simulink model "simulation"  (R2023a)
settings: Solver=VariableStepAuto  StartTime=0.0  StopTime=inf  RelTol=1e-3
values from neighbouring files (symbols this model uses):
  C_d = 0.1    [sim_script.m]
  C_l = 0.2    [parameters.m]
  fins_max_pos = deg2rad(15)    [parameters.m]
  fins_max_vel = deg2rad(180)    [parameters.m]
  g = 9.81    [parameters.m]    (also in sim_script.m)
  J_r = 0.000014703    (= 1.4703e-05)    [parameters.m]
  J_xx = 0.000834380    (= 0.00083438)    [parameters.m]
  J_yy = 0.000827389    [parameters.m]
  J_zz = 0.000150260    (= 0.00015026)    [parameters.m]
  K = lqr(A, B, Q, R)    [parameters.m]    (also in sim_script.m = lqr(A, B, Q, R, 0))
  K_t = 3.85756    [parameters.m]
  K_tau = 0.04249    [parameters.m]
  K_w = 0.0000014188    (= 1.4188e-06)    [parameters.m]    (also in sim_script.m = 1400)
  l = 0.04581 + 0.00625    (= 0.05206)    [parameters.m]    (also in sim_script.m = 0.1)
  m = 0.27765    [parameters.m]    (also in sim_script.m = 1)
  measurement_dt = 1/measurement_freq    (= 0.01)    [parameters.m]
  operating_point = [ ... (first row only)    [parameters.m]
  r = 0.06575    [parameters.m]    (also in sim_script.m = 0.05)
  variance_acc = 0.01    [parameters.m]
  variance_dst = 0.01    [parameters.m]
  variance_gyr = 0.01    [parameters.m]
  variance_mag = 0.01    [parameters.m]
undefined symbols (not defined in the file or in its folder): Discrete, throttle_max_rate, Time
libraries: sharedtransform x6, vrlib x4, commchan3 x4, matrix_library x2, shared6dof x1, ctrlSharedLib x1, sharedTrackingLibrary x1
settings Model: SimulationMode=accelerator  Creator=emozdzen  LastModifiedBy=emozdzen

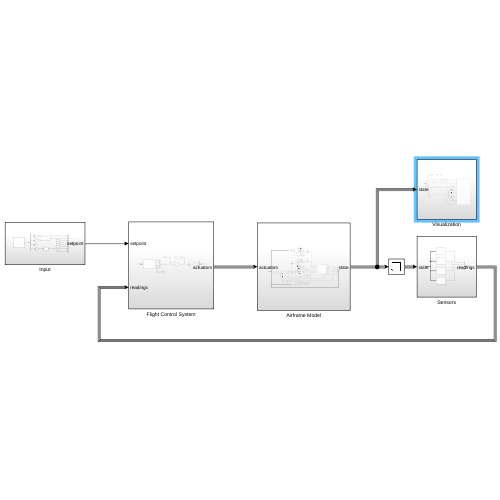
[thumbnail: Simulink's stored preview of the top-level diagram]
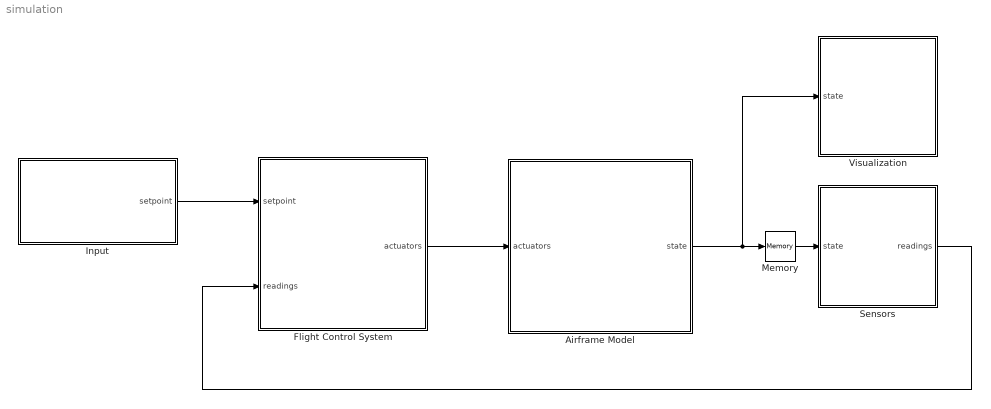
== system simulation ==
  Airframe Model : Subsystem
  Flight Control System : Subsystem
  Input : Subsystem
  Memory : Memory
  Sensors : Subsystem
  Visualization : Subsystem
  wires:
  Flight Control System/1(actuators) -> Airframe Model/1(actuators)
  Input/1(setpoint) -> Flight Control System/1(setpoint)
  Airframe Model/1(state) -> Visualization/1(state), Memory/1
  Sensors/1(readings) -> Flight Control System/2(readings)
  Memory/1 -> Sensors/1(state)

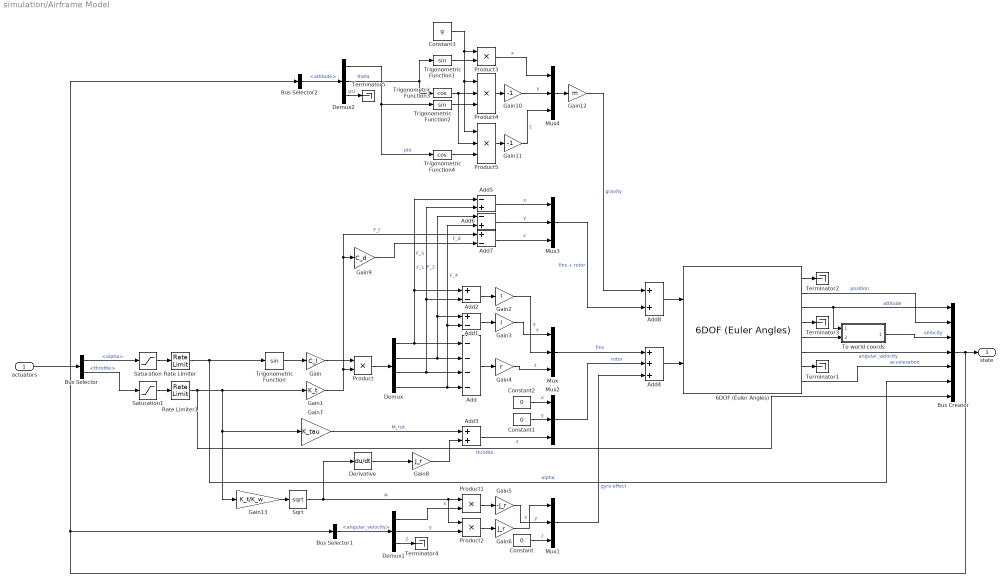
== system simulation/Airframe Model ==
  actuators : Inport
  6DOF (Euler Angles) : shared6dof/6DOF (Euler Angles)  units=Metric (MKS)  mtype=Fixed  rep=Euler Angles  xme_0=[0 0 0]  Vm_0=[0 0 0]  eul_0=[0 0 0]  pm_0=[0 0 0]  mass_0=m  mass_e=0.5  mass_f=2.0  inertia=[J_xx, 0, 0; 0, J_yy, 0; 0, 0, J_zz]  inertia_e=eye(3)  inertia_f=2*eye(3)  k_quat=1.0  vre_flag=on  abi_flag=off  aMode=0  xme_statename=''  Vm_statename=''  eul_statename=''  quat_statename=''  pm_statename=''  mass_statename=''
  Add : Sum  Inputs=----
  Add1 : Sum  Inputs=+-
  Add2 : Sum  Inputs=+-
  Add3 : Sum
  Add4 : Sum  Inputs=+++
  Add5 : Sum  Inputs=-+
  Add6 : Sum  Inputs=-+
  Add7 : Sum  Inputs=+-
  Add8 : Sum
  Bus Creator : BusCreator  Inputs=7
  Bus Selector : BusSelector  OutputSignals=alpha,throttle
  Bus Selector1 : BusSelector  OutputSignals=angular_velocity
  Bus Selector2 : BusSelector  OutputSignals=attitude
  Constant : Constant  Value=0
  Constant1 : Constant  Value=0
  Constant2 : Constant  Value=0
  Constant3 : Constant  Value=g
  Demux : Demux
  Demux1 : Demux  Outputs=3
  Demux2 : Demux  Outputs=3
  Derivative : Derivative
  Gain : Gain  Gain=C_l
  Gain1 : Gain  Gain=K_t
  Gain10 : Gain  Gain=-1
  Gain11 : Gain  Gain=-1
  Gain12 : Gain  Gain=m
  Gain13 : Gain  Gain=K_t/K_w
  Gain2 : Gain  Gain=l
  Gain3 : Gain  Gain=l
  Gain4 : Gain  Gain=r
  Gain5 : Gain  Gain=-J_r
  Gain6 : Gain  Gain=J_r
  Gain7 : Gain  Gain=K_tau
  Gain8 : Gain  Gain=J_r
  Gain9 : Gain  Gain=C_d
  Mux{,1..4} (5 alike) : Mux  Inputs=3
  Product{,1..3} (4 alike) : Product
  Product4 : Product  Inputs=3
  Product5 : Product  Inputs=3
  Rate Limiter : RateLimiter  RisingSlewLimit=fins_max_vel  FallingSlewLimit=-fins_max_vel  SampleTimeMode=inherited
  Rate Limiter1 : RateLimiter  RisingSlewLimit=throttle_max_rate  FallingSlewLimit=-throttle_max_rate  SampleTimeMode=inherited
  Saturation : Saturate  UpperLimit=fins_max_pos  LowerLimit=-fins_max_pos
  Saturation1 : Saturate  UpperLimit=1  LowerLimit=0
  Sqrt : Sqrt
  Terminator{1..5} (5 alike) : Terminator
  To world coords : Subsystem
  Trigonometric Function : Trigonometry
  Trigonometric Function1 : Trigonometry
  Trigonometric Function2 : Trigonometry
  Trigonometric Function3 : Trigonometry  Operator=cos
  Trigonometric Function4 : Trigonometry  Operator=cos
  state : Outport
  wires:
  actuators/1 -> Bus Selector/1
  Bus Creator/1 -> state/1, Bus Selector1/1, Bus Selector2/1
  6DOF (Euler Angles)/3 -> Bus Creator/1, To world coords/1(attitude)  "attitude"
  6DOF (Euler Angles)/6 -> Bus Creator/4  "angular_velocity"
  6DOF (Euler Angles)/2 -> Bus Creator/2  "position"
  6DOF (Euler Angles)/5 -> To world coords/2(in body)
  6DOF (Euler Angles)/8 -> Bus Creator/5  "acceleration"
  6DOF (Euler Angles)/7 -> Terminator1/1
  6DOF (Euler Angles)/1 -> Terminator2/1
  6DOF (Euler Angles)/4 -> Terminator3/1
  Bus Selector/1 -> Saturation/1  "<alpha>"
  Bus Selector/2 -> Saturation1/1  "<throttle>"
  Trigonometric Function/1 -> Gain/1
  Gain/1 -> Product/1
  Gain1/1 -> Add7/1, Gain9/1, Product/2  "F_t"
  Product/1 -> Demux/1
  Demux/1 -> Add5/1, Add2/1, Add/1  "F_1"
  Demux/2 -> Add6/1, Add1/1, Add/2  "F_2"
  Demux/3 -> Add2/2, Add5/2, Add/3  "F_3"
  Demux/4 -> Add6/2, Add1/2, Add/4  "F_4"
  Add2/1 -> Gain2/1
  Add1/1 -> Gain3/1
  Add/1 -> Gain4/1
  Gain3/1 -> Mux/1  "x"
  Gain2/1 -> Mux/2  "y"
  Gain4/1 -> Mux/3  "z"
  Mux/1 -> Add4/1  "fins"
  Bus Selector1/1 -> Demux1/1  "<angular_velocity>"
  Demux1/3 -> Terminator4/1  "z"
  Demux1/2 -> Product2/2  "y"
  Demux1/1 -> Product1/2  "x"
  Product1/1 -> Gain5/1
  Product2/1 -> Gain6/1
  Gain5/1 -> Mux1/2  "y"
  Gain6/1 -> Mux1/1  "x"
  Constant/1 -> Mux1/3  "z"
  Mux1/1 -> Add4/3  "gyro effect"
  Gain7/1 -> Add3/1  "M_rot"
  Constant1/1 -> Mux2/2  "y"
  Constant2/1 -> Mux2/1  "x"
  Mux2/1 -> Add4/2  "rotor"
  Add3/1 -> Mux2/3  "z"
  Derivative/1 -> Gain8/1
  Gain8/1 -> Add3/2
  Add4/1 -> 6DOF (Euler Angles)/2
  Bus Selector2/1 -> Demux2/1  "<attitude>"
  Gain9/1 -> Add7/2  "F_d"
  Add7/1 -> Mux3/3  "z"
  Add6/1 -> Mux3/2  "y"
  Add5/1 -> Mux3/1  "x"
  Mux3/1 -> Add8/2  "fins + rotor"
  Demux2/3 -> Terminator5/1  "psi"
  Demux2/2 -> Trigonometric Function1/1, Trigonometric Function3/1  "theta"
  Demux2/1 -> Trigonometric Function4/1, Trigonometric Function2/1  "phi"
  Trigonometric Function1/1 -> Product3/2
  Product3/1 -> Mux4/1  "x"
  Trigonometric Function2/1 -> Product4/3
  Trigonometric Function3/1 -> Product5/2, Product4/2
  Product4/1 -> Gain10/1
  Gain10/1 -> Mux4/2  "y"
  Mux4/1 -> Gain12/1
  Add8/1 -> 6DOF (Euler Angles)/1
  Trigonometric Function4/1 -> Product5/3
  Product5/1 -> Gain11/1
  Gain11/1 -> Mux4/3  "z"
  Saturation/1 -> Rate Limiter/1
  Saturation1/1 -> Rate Limiter1/1
  Rate Limiter/1 -> Bus Creator/6, Trigonometric Function/1  "alpha"
  Rate Limiter1/1 -> Gain7/1, Gain13/1, Gain1/1, Bus Creator/7  "throttle"
  Constant3/1 -> Product5/1, Product4/1, Product3/1
  Gain12/1 -> Add8/1  "gravity"
  To world coords/1(in world) -> Bus Creator/3  "velocity"
  Gain13/1 -> Sqrt/1
  Sqrt/1 -> Derivative/1, Product2/1, Product1/1  "w"

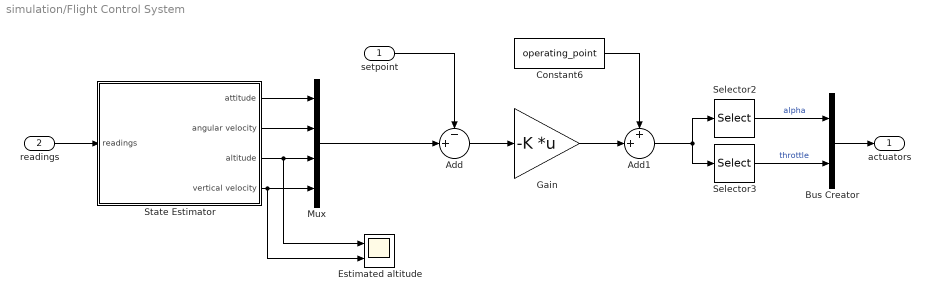
== system simulation/Flight Control System ==
  setpoint : Inport
  readings : Inport  Port=2
  Add : Sum  Inputs=-+|
  Add1 : Sum  Inputs=++|
  Bus Creator : BusCreator  Inputs=2
  Constant6 : Constant  Value=operating_point
  Estimated altitude : Scope  NumInputPorts=2
  Gain : Gain  Gain=-K  Multiplication=Matrix(K*u) (u vector)
  Mux : Mux
  Selector2 : Selector  InputPortWidth=5  IndexOptions=Index vector (dialog)  Indices=[1 2 3 4]  OutputSizes=1
  Selector3 : Selector  InputPortWidth=5  IndexOptions=Index vector (dialog)  Indices=[5]  OutputSizes=1
  State Estimator : Subsystem
  actuators : Outport
  wires:
  Bus Creator/1 -> actuators/1
  Add/1 -> Gain/1
  Gain/1 -> Add1/2
  Constant6/1 -> Add1/1
  Add1/1 -> Selector2/1, Selector3/1
  Selector2/1 -> Bus Creator/1  "alpha"
  setpoint/1 -> Add/1
  Selector3/1 -> Bus Creator/2  "throttle"
  readings/1 -> State Estimator/1(readings)
  State Estimator/1(attitude) -> Mux/1
  State Estimator/2(angular velocity) -> Mux/2
  State Estimator/3(altitude) -> Estimated altitude/1, Mux/3
  State Estimator/4(vertical velocity) -> Estimated altitude/2, Mux/4
  Mux/1 -> Add/2

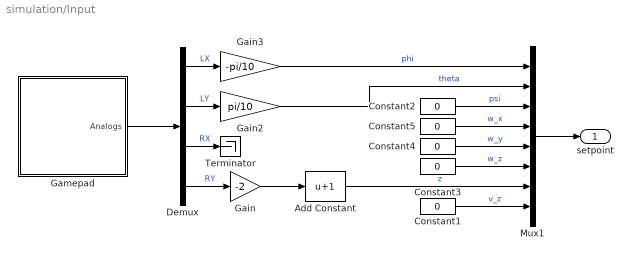
== system simulation/Input ==
  Add Constant : Bias  Bias=1  SaturateOnIntegerOverflow=off
  Constant{1..5} (5 alike) : Constant  Value=0
  Demux : Demux
  Gain : Gain  Gain=-2
  Gain2 : Gain  Gain=pi/10
  Gain3 : Gain  Gain=-pi/10
  Gamepad : Subsystem
  Mux1 : Mux  Inputs=8
  Terminator : Terminator
  setpoint : Outport
  wires:
  Gamepad/1(Analogs) -> Demux/1
  Demux/4 -> Gain/1  "RY"
  Demux/3 -> Terminator/1  "RX"
  Demux/2 -> Gain2/1  "LY"
  Demux/1 -> Gain3/1  "LX"
  Gain3/1 -> Mux1/1  "phi"
  Gain2/1 -> Mux1/2  "theta"
  Mux1/1 -> setpoint/1
  Constant1/1 -> Mux1/8  "v_z"
  Constant5/1 -> Mux1/4  "w_x"
  Constant4/1 -> Mux1/5  "w_y"
  Gain/1 -> Add Constant/1
  Constant3/1 -> Mux1/6  "w_z"
  Constant2/1 -> Mux1/3  "psi"
  Add Constant/1 -> Mux1/7  "z"

== system simulation/Sensors ==
  state : Inport
  Bus Creator : BusCreator  Inputs=4
  accelerometer : Subsystem
  gyroscope : Subsystem
  lidar : Subsystem
  magnetometer : Subsystem
  readings : Outport
  wires:
  Bus Creator/1 -> readings/1
  accelerometer/1(acceleration) -> Bus Creator/1  "acceleration"
  gyroscope/1(Out1) -> Bus Creator/2  "gyration"
  magnetometer/1(Out1) -> Bus Creator/3  "magnetic_field"
  lidar/1(distance) -> Bus Creator/4  "distance"
  state/1 -> lidar/1(state), magnetometer/1(state), accelerometer/1(state), gyroscope/1(state)

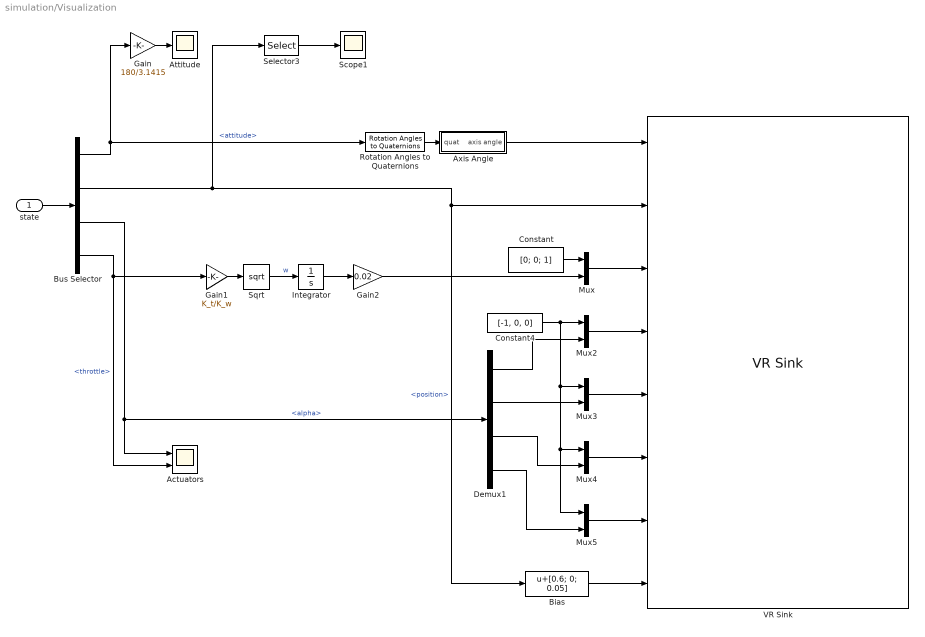
== system simulation/Visualization ==
  state : Inport
  Actuators : Scope  NumInputPorts=2
  Attitude : Scope
  "Axis Angle " : Subsystem
  Bias : Bias  Bias=[0.6; 0; 0.05]  SaturateOnIntegerOverflow=off
  Bus Selector : BusSelector  OutputSignals=attitude,position,alpha,throttle
  Constant : Constant  Value=[0; 0; 1]
  Constant4 : Constant  Value=[-1, 0, 0]
  Demux1 : Demux
  Gain : Gain  Gain=180/3.1415
  Gain1 : Gain  Gain=K_t/K_w
  Gain2 : Gain  Gain=0.02
  Integrator : Integrator
  Mux{,2..5} (5 alike) : Mux  Inputs=2
  Rotation Angles to Quaternions : sharedtransform/Rotation Angles to Quaternions  rotationOrder=XYZ  aMode=aMode
  Scope1 : Scope
  Selector3 : Selector  InputPortWidth=3  IndexOptions=Index vector (dialog)  Indices=[3]  OutputSizes=1
  Sqrt : Sqrt
  VR Sink : vrlib/VR Sink  InstantiateOnLoad=on  SampleTime=0.02  ViewEnable=on  RemoteChange=off  RemoteView=off  FieldsWritten=body.rotation.4.1.1.double#body.translation.3.1.1.double#rotor.rotation.4.1.1.double#fin1.rotation.4.1.1.double#fin2.rotation.4.1.1.double#fin3.rotation.4.1.1.double#fin4.rotation.4.1.1.double#follower.position.3.1.1.double  WorldFileName=word.wrl  AutoView=off  VideoDimensions=[]  AllowVariableSize=off  FigureProperties="{'Position', 'Name', 'Viewpoint', 'CameraBound', 'CameraDirection', 'CameraPosition', 'CameraUpVector', 'ZoomFactor', 'Antialiasing', 'Headlight', 'Lighting', 'NavPanel', 'Sound', 'StatusBar', 'Stereo3D', 'Stereo3DCameraOffset', 'Stereo3DHIT', 'ToolBar', 'Textures', 'Transparency', 'Triad', 'Wireframe', 'NavZones', 'NavMode', 'NavSpeed', 'CaptureFileFormat', 'CaptureFileName', 'Record2DCompressMethod', 'Record2DCompressQuality', 'Record2D', 'Record2DFileName', 'Record2DFPS'; [2.3870000000000000e+03   3.7500000000000000e+02   5.7600000000000000e+02   3.5000000000000000e+02], '', 'follower', 'on', [0.0000000000000000e+00   0.0000000000000000e+00  -1.0000000000000000e+00], [0.0000000000000000e+00   0.0000000000000000e+00   0.0000000000000000e+00], [0.0000000000000000e+00   1.0000000000000000e+00   0.0000000000000000e+00], [1.0000000000000000e+00], 'on', 'on', 'on', 'halfbar', 'on', 'on', 'off', [1.0000000149011612e-01], [0.0000000000000000e+00], 'on', 'on', 'on', 'none', 'off', 'off', 'fly', 'normal', 'tif', '%f_anim_%n.tif', 'auto', [7.5000000000000000e+01], 'off', '%f_anim_%n.avi', 'auto'}"
  wires:
  state/1 -> Bus Selector/1
  Bus Selector/1 -> Rotation Angles to Quaternions/1, Gain/1  "<attitude>"
  Bus Selector/2 -> VR Sink/2, Bias/1, Selector3/1  "<position>"
  Demux1/4 -> Mux5/2
  Demux1/1 -> Mux2/2
  Demux1/2 -> Mux3/2
  Demux1/3 -> Mux4/2
  Rotation Angles to Quaternions/1 -> "Axis Angle "/1(quat)
  Bus Selector/3 -> Actuators/1, Demux1/1  "<alpha>"
  Bus Selector/4 -> Actuators/2, Gain1/1  "<throttle>"
  Selector3/1 -> Scope1/1
  Gain/1 -> Attitude/1
  Integrator/1 -> Gain2/1
  Gain1/1 -> Sqrt/1
  Sqrt/1 -> Integrator/1  "w"
  Gain2/1 -> Mux/2
  Constant/1 -> Mux/1
  "Axis Angle "/1(axis angle) -> VR Sink/1
  Mux/1 -> VR Sink/3
  Bias/1 -> VR Sink/8
  Mux2/1 -> VR Sink/4
  Mux3/1 -> VR Sink/5
  Mux4/1 -> VR Sink/6
  Mux5/1 -> VR Sink/7
  Constant4/1 -> Mux5/1, Mux4/1, Mux3/1, Mux2/1

== system simulation/Airframe Model/To world coords ==
  attitude : Inport
  in body : Inport  Port=2
  Product : Product  Multiplication=Matrix(*)
  Rotation Angles to Direction Cosine Matrix : sharedtransform/Rotation Angles to Direction Cosine Matrix  rotationOrder=XYZ  aMode=aMode
  Transpose : matrix_library/Transpose
  in world : Outport
  wires:
  Product/1 -> in world/1
  Rotation Angles to Direction Cosine Matrix/1 -> Transpose/1
  in body/1 -> Product/2
  attitude/1 -> Rotation Angles to Direction Cosine Matrix/1
  Transpose/1 -> Product/1

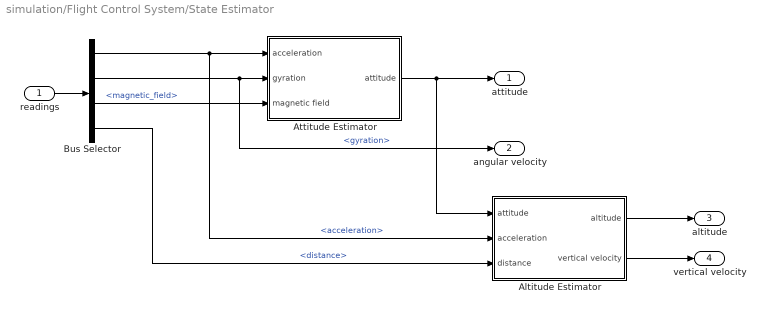
== system simulation/Flight Control System/State Estimator ==
  readings : Inport
  Altitude Estimator : Subsystem
  Attitude Estimator : Subsystem
  Bus Selector : BusSelector  OutputSignals=acceleration,gyration,magnetic_field,distance
  attitude : Outport
  angular velocity : Outport  Port=2
  altitude : Outport  Port=3
  vertical velocity : Outport  Port=4
  wires:
  readings/1 -> Bus Selector/1
  Attitude Estimator/1(attitude) -> attitude/1, Altitude Estimator/1(attitude)
  Bus Selector/1 -> Altitude Estimator/2(acceleration), Attitude Estimator/1(acceleration)  "<acceleration>"
  Bus Selector/2 -> angular velocity/1, Attitude Estimator/2(gyration)  "<gyration>"
  Bus Selector/3 -> Attitude Estimator/3(magnetic field)  "<magnetic_field>"
  Altitude Estimator/1(altitude) -> altitude/1
  Altitude Estimator/2(vertical velocity) -> vertical velocity/1
  Bus Selector/4 -> Altitude Estimator/3(distance)  "<distance>"

== system simulation/Input/Gamepad ==
  Display : Display
  Display1 : Display
  Joystick Input : vrlib/Joystick Input  joyid=1  adjustports=on  forcefeed=off
  Selector : Selector  InputPortWidth=8  IndexOptions=Index vector (dialog)  Indices=[1 2 4 5]  OutputSizes=1
  Analogs : Outport
  wires:
  Joystick Input/2 -> Display1/1
  Joystick Input/1 -> Selector/1, Display/1
  Selector/1 -> Analogs/1

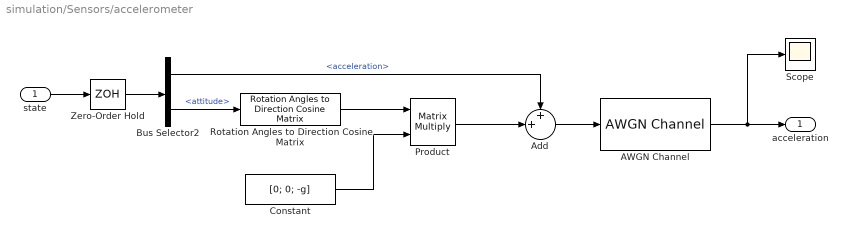
== system simulation/Sensors/accelerometer ==
  state : Inport
  AWGN Channel : commchan3/AWGN Channel  LegacyMode=off  NoiseMethod=Variance  noiseMode="Signal to noise ratio  (SNR)"  EbNo=10  EsNo=10  SNR=10  BitsPerSymbol=1  SignalPower=1  SamplesPerSymbol=1  SymbolPeriod=1  VarianceSource=Parameter  Variance=variance_acc  RandomStream=Global stream  Seed=67  SimulateUsing=Code generation
  Add : Sum  Inputs=++|
  Bus Selector2 : BusSelector  OutputSignals=acceleration,attitude
  Constant : Constant  Value=[0; 0; -g]
  Product : Product  Multiplication=Matrix(*)
  Rotation Angles to Direction Cosine Matrix : sharedtransform/Rotation Angles to Direction Cosine Matrix  rotationOrder=XYZ  aMode=aMode
  Scope : Scope
  Zero-Order Hold : ZeroOrderHold  SampleTime=measurement_dt
  acceleration : Outport
  wires:
  state/1 -> Zero-Order Hold/1
  Bus Selector2/2 -> Rotation Angles to Direction Cosine Matrix/1  "<attitude>"
  Rotation Angles to Direction Cosine Matrix/1 -> Product/1
  Constant/1 -> Product/2
  Product/1 -> Add/2
  Bus Selector2/1 -> Add/1  "<acceleration>"
  Add/1 -> AWGN Channel/1
  Zero-Order Hold/1 -> Bus Selector2/1
  AWGN Channel/1 -> Scope/1, acceleration/1

== system simulation/Sensors/gyroscope ==
  state : Inport
  AWGN Channel : commchan3/AWGN Channel  LegacyMode=off  NoiseMethod=Variance  noiseMode="Signal to noise ratio  (SNR)"  EbNo=10  EsNo=10  SNR=10  BitsPerSymbol=1  SignalPower=1  SamplesPerSymbol=1  SymbolPeriod=1  VarianceSource=Parameter  Variance=variance_gyr  RandomStream=Global stream  Seed=67  SimulateUsing=Code generation
  Bus Selector : BusSelector  OutputSignals=angular_velocity
  Scope : Scope
  Zero-Order Hold : ZeroOrderHold  SampleTime=measurement_dt
  Out1 : Outport
  wires:
  state/1 -> Zero-Order Hold/1
  Bus Selector/1 -> AWGN Channel/1  "<angular_velocity>"
  Zero-Order Hold/1 -> Bus Selector/1
  AWGN Channel/1 -> Scope/1, Out1/1

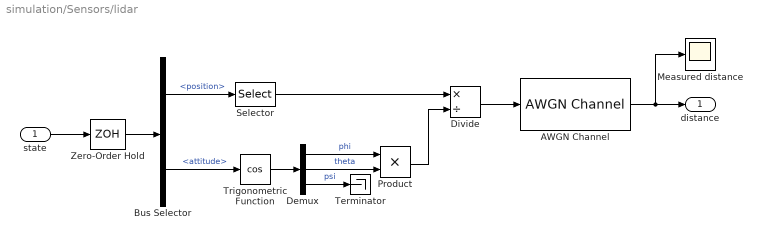
== system simulation/Sensors/lidar ==
  state : Inport
  AWGN Channel : commchan3/AWGN Channel  LegacyMode=off  NoiseMethod=Variance  noiseMode="Signal to noise ratio  (SNR)"  EbNo=10  EsNo=10  SNR=10  BitsPerSymbol=1  SignalPower=1  SamplesPerSymbol=1  SymbolPeriod=1  VarianceSource=Parameter  Variance=variance_dst  RandomStream=Global stream  Seed=67  SimulateUsing=Code generation
  Bus Selector : BusSelector  OutputSignals=position,attitude
  Demux : Demux  Outputs=3
  Divide : Product  Inputs=*/
  Measured distance : Scope
  Product : Product
  Selector : Selector  InputPortWidth=3  IndexOptions=Index vector (dialog)  Indices=[3]  OutputSizes=1
  Terminator : Terminator
  Trigonometric Function : Trigonometry  Operator=cos
  Zero-Order Hold : ZeroOrderHold  SampleTime=measurement_dt
  distance : Outport
  wires:
  state/1 -> Zero-Order Hold/1
  Bus Selector/1 -> Selector/1  "<position>"
  Bus Selector/2 -> Trigonometric Function/1  "<attitude>"
  Selector/1 -> Divide/1
  Demux/3 -> Terminator/1  "psi"
  Demux/2 -> Product/2  "theta"
  Demux/1 -> Product/1  "phi"
  Trigonometric Function/1 -> Demux/1
  Product/1 -> Divide/2
  AWGN Channel/1 -> Measured distance/1, distance/1
  Zero-Order Hold/1 -> Bus Selector/1
  Divide/1 -> AWGN Channel/1

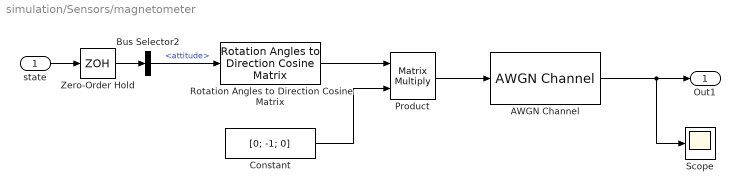
== system simulation/Sensors/magnetometer ==
  state : Inport
  AWGN Channel : commchan3/AWGN Channel  LegacyMode=off  NoiseMethod=Variance  noiseMode="Signal to noise ratio  (SNR)"  EbNo=10  EsNo=10  SNR=10  BitsPerSymbol=1  SignalPower=1  SamplesPerSymbol=1  SymbolPeriod=1  VarianceSource=Parameter  Variance=variance_mag  RandomStream=Global stream  Seed=67  SimulateUsing=Code generation
  Bus Selector2 : BusSelector  OutputSignals=attitude
  Constant : Constant  Value=[0; -1; 0]
  Product : Product  Multiplication=Matrix(*)
  Rotation Angles to Direction Cosine Matrix : sharedtransform/Rotation Angles to Direction Cosine Matrix  rotationOrder=XYZ  aMode=aMode
  Scope : Scope
  Zero-Order Hold : ZeroOrderHold  SampleTime=measurement_dt
  Out1 : Outport
  wires:
  Bus Selector2/1 -> Rotation Angles to Direction Cosine Matrix/1  "<attitude>"
  Constant/1 -> Product/2
  Rotation Angles to Direction Cosine Matrix/1 -> Product/1
  state/1 -> Zero-Order Hold/1
  Product/1 -> AWGN Channel/1
  Zero-Order Hold/1 -> Bus Selector2/1
  AWGN Channel/1 -> Scope/1, Out1/1

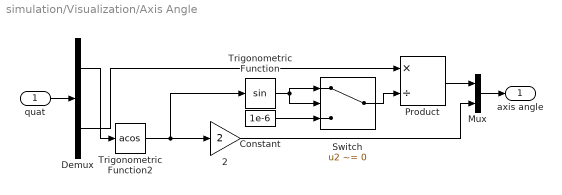
== system simulation/Visualization/Axis Angle  ==
  quat : Inport
  2 : Gain  Gain=2  SaturateOnIntegerOverflow=on  OutDataTypeStr=Inherit: Same as input  ParamDataTypeStr=Inherit: Same as input
  Constant : Constant  Value=1e-6
  Demux : Demux  Outputs=[1 3 ]
      settings: DisplayOption=none
  Mux : Mux  Inputs=2
  Product : Product  Inputs=*/  InputSameDT=on  SaturateOnIntegerOverflow=on  OutDataTypeStr=Inherit: Same as first input
  Switch : Switch  Criteria=u2 ~= 0  SaturateOnIntegerOverflow=off  InputSameDT=off
  Trigonometric Function : Trigonometry
  Trigonometric Function2 : Trigonometry  Operator=acos
  axis angle : Outport  VectorParamsAs1DForOutWhenUnconnected=off
  wires:
  Demux/1 -> Trigonometric Function2/1
  Demux/2 -> Product/1
  Mux/1 -> axis angle/1
  Product/1 -> Mux/1
  2/1 -> Mux/2
  Trigonometric Function/1 -> Switch/1, Switch/2
  Trigonometric Function2/1 -> Trigonometric Function/1, 2/1
  quat/1 -> Demux/1
  Constant/1 -> Switch/3
  Switch/1 -> Product/2

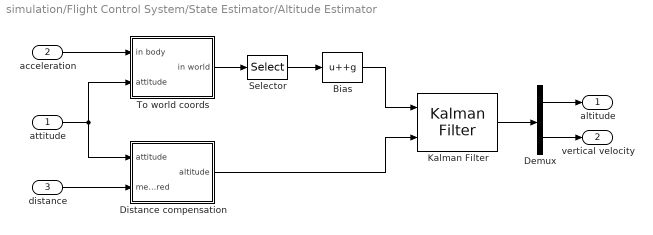
== system simulation/Flight Control System/State Estimator/Altitude Estimator ==
  attitude : Inport
  acceleration : Inport  Port=2
  distance : Inport  Port=3
  Bias : Bias  Bias=+g  SaturateOnIntegerOverflow=off
  Demux : Demux  Outputs=2
  Distance compensation : Subsystem
  Kalman Filter : ctrlSharedLib/Kalman Filter  TimeDomain=Discrete-Time  UseCurrentEstimator=on  ModelSource=Individual A, B, C, D matrices  ModelSourceVariable=ss(0.95,1,1,0,1)  A=[1, measurement_dt; 0, 1;]  B=[0.5*measurement_dt*measurement_dt; measurement_dt;]  C=[1, 0]  D=0  NumberOfStates=1  NumberOfInputs=1  NumberOfOutputs=1  InitialEstimateSource=Dialog  X0=[0; 0;]  P0=10  UseK=off  UseGH=off  NumberOfProcessNoiseInputs=1  G=1  TimeInvariantG=on  H=0  TimeInvariantH=on  Q=variance_acc  TimeInvariantQ=on  R=variance_dst  TimeInvariantR=on  N=0  TimeInvariantN=on  AddInputPort=on  AddEnablePort=off  OutputEstimatedY=off  OutputP=off  Ts=measurement_dt
  Selector : Selector  InputPortWidth=3  IndexOptions=Index vector (dialog)  Indices=[3]  OutputSizes=1
  To world coords : Subsystem
  altitude : Outport
  vertical velocity : Outport  Port=2
  wires:
  Distance compensation/1(altitude) -> Kalman Filter/2
  To world coords/1(in world) -> Selector/1
  Selector/1 -> Bias/1
  Kalman Filter/1 -> Demux/1
  Demux/2 -> vertical velocity/1
  Demux/1 -> altitude/1
  distance/1 -> Distance compensation/2(measured)
  acceleration/1 -> To world coords/1(in body)
  attitude/1 -> Distance compensation/1(attitude), To world coords/2(attitude)
  Bias/1 -> Kalman Filter/1

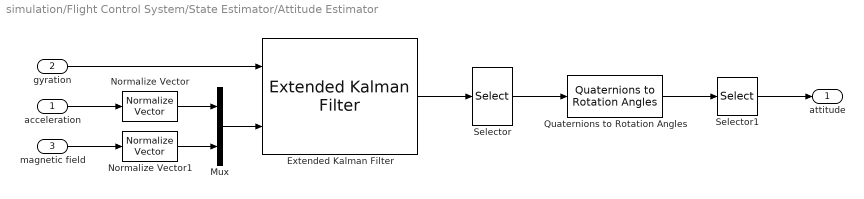
== system simulation/Flight Control System/State Estimator/Attitude Estimator ==
  acceleration : Inport
  gyration : Inport  Port=2
  magnetic field : Inport  Port=3
  Extended Kalman Filter : sharedTrackingLibrary/Extended Kalman Filter  StateTransitionFcn=AttitudeStateTransitionFcn  HasStateTransitionJacobianFcn=off  HasAdditiveProcessNoise=Additive  ProcessNoise=eye(7)*0.001  HasTimeVaryingProcessNoise=off  HasStateTransitionFcnExtraArgument=1  InitialState=[0; -1; 0; 0; 0; 0; 0]  InitialStateCovariance=1e+6  MeasurementFcn1=AttitudeMeasurementFcn  HasMeasurementJacobianFcn1=off  HasMeasurementEnablePort1=off  HasAdditiveMeasurementNoise1=Additive  MeasurementNoise1=diag([variance_acc, variance_acc, variance_acc, variance_mag, variance_mag, variance_mag])  HasTimeVaryingMeasurementNoise1=off  HasMeasurementFcnExtraArgument1=0  HasMeasurementWrapping1=off  MeasurementFcn2=myMeasurementFcn  HasMeasurementJacobianFcn2=off  HasMeasurementEnablePort2=off  HasAdditiveMeasurementNoise2=Additive  MeasurementNoise2=1  HasTimeVaryingMeasurementNoise2=off  HasMeasurementFcnExtraArgument2=0  HasMeasurementWrapping2=off  MeasurementFcn3=myMeasurementFcn  HasMeasurementJacobianFcn3=off  HasMeasurementEnablePort3=off  HasAdditiveMeasurementNoise3=Additive  MeasurementNoise3=1  HasTimeVaryingMeasurementNoise3=off  HasMeasurementFcnExtraArgument3=0  HasMeasurementWrapping3=off  MeasurementFcn4=myMeasurementFcn  HasMeasurementJacobianFcn4=off  HasMeasurementEnablePort4=off  HasAdditiveMeasurementNoise4=Additive  MeasurementNoise4=1  HasTimeVaryingMeasurementNoise4=off  HasMeasurementFcnExtraArgument4=0  HasMeasurementWrapping4=off  MeasurementFcn5=myMeasurementFcn  HasMeasurementJacobianFcn5=off  HasMeasurementEnablePort5=off  HasAdditiveMeasurementNoise5=Additive  MeasurementNoise5=1  HasTimeVaryingMeasurementNoise5=off  HasMeasurementFcnExtraArgument5=0  HasMeasurementWrapping5=off  EnableMultirate=off  StateTransitionFcnSampleTime=1  MeasurementFcn1SampleTime=1  MeasurementFcn2SampleTime=1  MeasurementFcn3SampleTime=1  MeasurementFcn4SampleTime=1  MeasurementFcn5SampleTime=1  UseCurrentEstimator=on  OutputStateCovariance=off  DataType=double  SampleTime=measurement_dt  NumberOfMeasurements=1
  Mux : Mux  Inputs=2
  Normalize Vector : vrlib/Utilities/Normalize Vector  maxzero=0
  Normalize Vector1 : vrlib/Utilities/Normalize Vector  maxzero=0
  Quaternions to Rotation Angles : sharedtransform/Quaternions to Rotation Angles  rotationOrder=ZYX  aMode=aMode
  Selector : Selector  InputPortWidth=7  IndexOptions=Index vector (dialog)  Indices=[1 2 3 4]  OutputSizes=1
  Selector1 : Selector  InputPortWidth=3  IndexOptions=Index vector (dialog)  Indices=[3 2 1]  OutputSizes=1
  attitude : Outport
  wires:
  gyration/1 -> Extended Kalman Filter/1
  acceleration/1 -> Normalize Vector/1
  magnetic field/1 -> Normalize Vector1/1
  Mux/1 -> Extended Kalman Filter/2
  Extended Kalman Filter/1 -> Selector/1
  Selector/1 -> Quaternions to Rotation Angles/1
  Quaternions to Rotation Angles/1 -> Selector1/1
  Selector1/1 -> attitude/1
  Normalize Vector/1 -> Mux/1
  Normalize Vector1/1 -> Mux/2

== system simulation/Flight Control System/State Estimator/Altitude Estimator/Distance compensation ==
  attitude : Inport
  measured : Inport  Port=2
  Demux : Demux  Outputs=3
  Product : Product  Inputs=3
  Terminator : Terminator
  Trigonometric Function : Trigonometry  Operator=cos
  altitude : Outport
  wires:
  attitude/1 -> Trigonometric Function/1
  Trigonometric Function/1 -> Demux/1
  Demux/3 -> Terminator/1
  Demux/2 -> Product/3
  Demux/1 -> Product/2
  measured/1 -> Product/1
  Product/1 -> altitude/1

== system simulation/Flight Control System/State Estimator/Altitude Estimator/To world coords ==
  in body : Inport
  attitude : Inport  Port=2
  Product : Product  Multiplication=Matrix(*)
  Rotation Angles to Direction Cosine Matrix : sharedtransform/Rotation Angles to Direction Cosine Matrix  rotationOrder=XYZ  aMode=aMode
  Transpose : matrix_library/Transpose
  in world : Outport
  wires:
  attitude/1 -> Rotation Angles to Direction Cosine Matrix/1
  in body/1 -> Product/2
  Rotation Angles to Direction Cosine Matrix/1 -> Transpose/1
  Transpose/1 -> Product/1
  Product/1 -> in world/1
